simulink model "holiday2"  (R2019a)
settings: Solver=VariableStepAuto  StartTime=0.0  StopTime=10.0  RelTol=1e-3
settings Model: Creator=Aditya  LastModifiedBy=Aditya

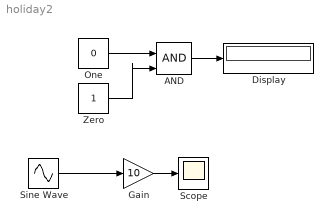
== system holiday2 ==
  AND : Logic  IconShape=distinctive  AllPortsSameDT=off  OutDataTypeStr=boolean
  Display : Display
  Gain : Gain  Gain=10
  One : Constant  Value=0  OutDataTypeStr=Inherit: Inherit via back propagation
  Scope : Scope
  Sine Wave : Sin  SampleTime=0
  Zero : Constant  OutDataTypeStr=Inherit: Inherit via back propagation
  wires:
  Sine Wave/1 -> Gain/1
  Gain/1 -> Scope/1
  AND/1 -> Display/1
  One/1 -> AND/1
  Zero/1 -> AND/2
